simulink model "Posture_Regulation_NO_Singularity_ROS"  (R2022b)
settings: Solver=FixedStepAuto  StartTime=0.0  StopTime=80  FixedStep=0.02  MaxStep=0.1  RelTol=1e-3
undefined symbols (not defined in the file): theta_f, unicycle, X, x_f, Y, y_f
libraries: simulink_extras x4, robotlib x3
settings Model: Creator=Musta  LastModifiedBy=mustacchim
settings OptimizationCC: EnhancedBackFolding=on  PassReuseOutputArgsAs=Individual arguments  ZeroExternalMemoryAtStartup=off  ZeroInternalMemoryAtStartup=off  MaxStackSize=64  OptimizeBlockOrder=speed  DifferentSizesBufferReuse=on  OptimizationCustomize=off  EfficientTunableParamExpr=on
settings DebuggingCC: ParameterTunabilityLossMsg=error
settings HardwareCC: ProdBitPerPointer=32  ProdBitPerSizeT=32  ProdBitPerPtrDiffT=32  ProdLargestAtomicFloat=None  ProdIntDivRoundTo=Undefined  ProdEndianess=Unspecified  ProdWordSize=32  ProdHWDeviceType=Generic->Unspecified (assume 32-bit Generic)
settings SFSimCC: MATLABDynamicMemAlloc=off
settings RTWCC: Description=Embedded Coder  SystemTargetFile=ert.tlc  HardwareBoard=Robot Operating System (ROS)  TLCOptions="-aInlineSetEventsForThisBaseRateFcn=TLC_FALSE -aSuppressMultiTaskScheduler=TLC_FALSE  -aRateBasedStepFcn=0"  TemplateMakefile=ert_default_tmf  Toolchain=Catkin  TargetLang=C++
settings CodeAppCC: ForceParamTrailComments=on  IgnoreCustomStorageClasses=off  OperatorAnnotations=on  SimulinkDataObjDesc=on  SFDataObjDesc=on  InsertBlockDesc=on

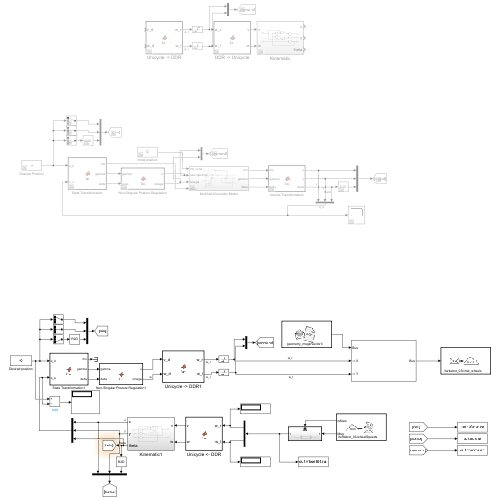
[thumbnail: Simulink's stored preview of the top-level diagram]
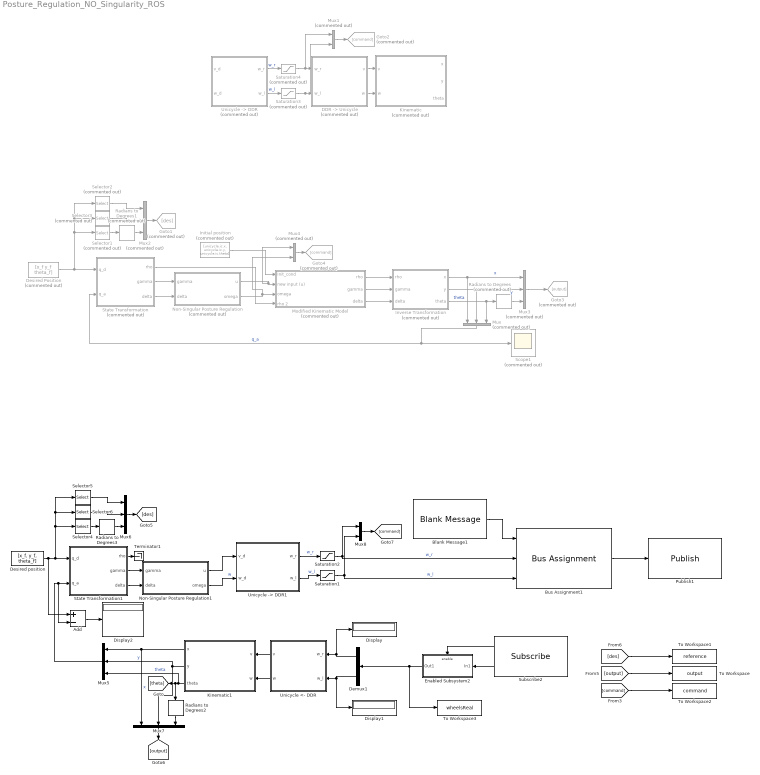
== system Posture_Regulation_NO_Singularity_ROS ==
  " DDR -> Unicycle " : MATLAB Function  Commented=on  TreatAsAtomicUnit=on
  Add : Sum  Inputs=+-
  Blank Message1 : robotlib/Blank Message  messageClass=Message  entityType=geometry_msgs/Vector3  messageType=geometry_msgs/Vector3  SampleTime=0.02  legacyBusStruct=off
      settings: LibrarySourceBlock=roslib/ROS/Blank Message
  Bus Assignment1 : BusAssignment  AssignedSignals=X,Y
  Demux1 : Demux  Outputs=2
  Desired Position : Constant  Commented=on  Value=[x_f y_f theta_f]
  Desired position : Constant  Value=[x_f, y_f, theta_f]
  Display : Display
  Display1 : Display
  Display2 : Display
  Enabled Subsystem2 : Subsystem  TreatAsAtomicUnit=on
  Goto1 : Goto  Commented=on  GotoTag=des
  Goto2 : Goto  Commented=on  GotoTag=command
  Goto3 : Goto  Commented=on  GotoTag=output
  Goto4 : Goto  Commented=on  GotoTag=command
  Initial position : Constant  Commented=on  Value=[unicycle.ic.x, unicycle.ic.y, unicycle.ic.theta]
  Inverse Transformation : MATLAB Function  Commented=on  TreatAsAtomicUnit=on
  Kinematic : Subsystem  Commented=on
  Kinematic1 : Subsystem
  Modified Kinematic Model : Subsystem  Commented=on
  Mux : Mux  Commented=on  Inputs=3
  Mux1 : Mux  Commented=on  Inputs=2
  Mux2 : Mux  Commented=on  Inputs=3
  Mux3 : Mux  Commented=on  Inputs=3
  Mux4 : Mux  Commented=on  Inputs=2
  Mux5 : Mux  Inputs=3
  Mux6 : Mux  Inputs=3
  Mux7 : Mux  Inputs=3
  Mux8 : Mux  Inputs=2
  Non-Singular Posture Regulation : MATLAB Function  Commented=on  TreatAsAtomicUnit=on
  Non-Singular Posture Regulation1 : MATLAB Function  TreatAsAtomicUnit=on
  Publish1 : robotlib/Publish  topicSource=Select from ROS network  topic=/turtlebot_03/cmd_wheels  messageType=geometry_msgs/Vector3  legacyBusStruct=off  messageQueueLength=1
      settings: LibrarySourceBlock=roslib/ROS/Publish
  Radians to Degrees : simulink_extras/Transformations/Radians to Degrees  Commented=on
  Radians to Degrees1 : simulink_extras/Transformations/Radians to Degrees  Commented=on
  Radians to Degrees2 : simulink_extras/Transformations/Radians to Degrees
  Radians to Degrees3 : simulink_extras/Transformations/Radians to Degrees
  Saturation1 : Saturate  UpperLimit=unicycle.omegaWheelMax  LowerLimit=unicycle.omegaWheelMin
  Saturation2 : Saturate  UpperLimit=unicycle.omegaWheelMax  LowerLimit=unicycle.omegaWheelMin
  Saturation3 : Saturate  Commented=on  UpperLimit=unicycle.omegaWheelMax  LowerLimit=unicycle.omegaWheelMin
  Saturation4 : Saturate  Commented=on  UpperLimit=unicycle.omegaWheelMax  LowerLimit=unicycle.omegaWheelMin
  Scope1 : Scope  Commented=on
  Selector1 : Selector  Commented=on  InputPortWidth=3  IndexOptions=Index vector (dialog)  Indices=3  OutputSizes=1
  Selector2 : Selector  Commented=on  InputPortWidth=3  IndexOptions=Index vector (dialog)  Indices=1  OutputSizes=1
  Selector3 : Selector  Commented=on  InputPortWidth=3  IndexOptions=Index vector (dialog)  Indices=2  OutputSizes=1
  Selector4 : Selector  InputPortWidth=3  IndexOptions=Index vector (dialog)  Indices=3  OutputSizes=1
  Selector5 : Selector  InputPortWidth=3  IndexOptions=Index vector (dialog)  Indices=1  OutputSizes=1
  Selector6 : Selector  InputPortWidth=3  IndexOptions=Index vector (dialog)  Indices=2  OutputSizes=1
  State Transformation : MATLAB Function  Commented=on  TreatAsAtomicUnit=on
  State Transformation1 : MATLAB Function  TreatAsAtomicUnit=on
  Subscribe2 : robotlib/Subscribe  topicSource=Select from ROS network  topic=/turtlebot_03/wheelSpeeds  messageType=geometry_msgs/Vector3  SampleTime=0.02  legacyBusStruct=off  messageQueueLength=1
      settings: LibrarySourceBlock=roslib/ROS/Subscribe
  Terminator1 : Terminator
  To Workspace : ToWorkspace  VariableName=output  SaveFormat=Structure With Time  SampleTime=-1
  To Workspace1 : ToWorkspace  VariableName=reference  SaveFormat=Structure With Time  SampleTime=-1
  To Workspace2 : ToWorkspace  VariableName=command  SaveFormat=Structure With Time  SampleTime=-1
  To Workspace3 : ToWorkspace  VariableName=wheelsReal  SaveFormat=Structure With Time  SampleTime=-1
  "Unicycle -> DDR" : MATLAB Function  Commented=on  TreatAsAtomicUnit=on
  "Unicycle -> DDR1" : MATLAB Function  TreatAsAtomicUnit=on
  Unicycle <- DDR : MATLAB Function  TreatAsAtomicUnit=on
  wires:
  [command] -> To Workspace2/1
  [des] -> To Workspace1/1
  [output] -> To Workspace/1
  Selector2/1 -> Mux2/1
  Mux/1 -> Scope1/1, State Transformation/2(q_a)  "q_a"
  Selector3/1 -> Mux2/2
  Inverse Transformation/1(x) -> Mux/1, Mux3/1  "x"
  Desired Position/1 -> Selector2/1, Selector3/1, Selector1/1, State Transformation/1(q_d)
  Inverse Transformation/3(theta) -> Mux/3, Radians to Degrees/1  "theta"
  Radians to Degrees/1 -> Mux3/3
  Inverse Transformation/2(y) -> Mux3/2, Mux/2  "y"
  Modified Kinematic Model/3(delta) -> Inverse Transformation/3(delta)
  Mux2/1 -> Goto1/1
  State Transformation/1(rho) -> Modified Kinematic Model/4(rho 2)
  Radians to Degrees1/1 -> Mux2/3
  Selector1/1 -> Radians to Degrees1/1
  Modified Kinematic Model/1(rho) -> Inverse Transformation/1(rho)
  Mux4/1 -> Goto4/1
  Modified Kinematic Model/2(gamma) -> Inverse Transformation/2(gamma)
  State Transformation/3(delta) -> Non-Singular Posture Regulation/2(delta)
  Initial position/1 -> Modified Kinematic Model/1(Init_cond)
  Non-Singular Posture Regulation/1(u) -> Modified Kinematic Model/2(new input (u)), Mux4/1
  Mux3/1 -> Goto3/1
  Non-Singular Posture Regulation/2(omega) -> Mux4/2, Modified Kinematic Model/3(omega)
  State Transformation/2(gamma) -> Non-Singular Posture Regulation/1(gamma)
  "Unicycle -> DDR"/2(w_l) -> Saturation3/1  "w_l"
  " DDR -> Unicycle "/1(v) -> Kinematic/1(v)
  "Unicycle -> DDR"/1(w_r) -> Saturation4/1  "w_r"
  Mux1/1 -> Goto2/1
  Saturation4/1 -> Mux1/1, " DDR -> Unicycle "/1(w_r)
  Saturation3/1 -> Mux1/2, " DDR -> Unicycle "/2(w_l)
  " DDR -> Unicycle "/2(w) -> Kinematic/2(w)
  Radians to Degrees2/1 -> Mux7/3
  Bus Assignment1/1 -> Publish1/1
  Selector4/1 -> Radians to Degrees3/1
  Subscribe2/2 -> Enabled Subsystem2/1(In1)
  State Transformation1/2(gamma) -> Non-Singular Posture Regulation1/1(gamma)
  Demux1/2 -> Display1/1, Unicycle <- DDR/2(w_l)
  Saturation2/1 -> Bus Assignment1/2, Mux8/1  "w_r"
  Unicycle <- DDR/1(v) -> Kinematic1/1(v)
  Mux6/1 -> [des]
  "Unicycle -> DDR1"/1(w_r) -> Saturation2/1  "w_r"
  Non-Singular Posture Regulation1/1(u) -> "Unicycle -> DDR1"/1(v_d)
  Kinematic1/3(theta) -> Mux5/3, Radians to Degrees2/1, [theta]  "theta"
  Saturation1/1 -> Bus Assignment1/3, Mux8/2  "w_l"
  State Transformation1/1(rho) -> Terminator1/1
  Demux1/1 -> Display/1, Unicycle <- DDR/1(w_r)
  Selector6/1 -> Mux6/2
  Mux7/1 -> [output]
  "Unicycle -> DDR1"/2(w_l) -> Saturation1/1  "w_l"
  Radians to Degrees3/1 -> Mux6/3
  Blank Message1/1 -> Bus Assignment1/1
  Kinematic1/2(y) -> Mux7/2, Mux5/2  "y"
  Unicycle <- DDR/2(w) -> Kinematic1/2(w)
  Mux5/1 -> Add/2, State Transformation1/2(q_a)
  Non-Singular Posture Regulation1/2(omega) -> "Unicycle -> DDR1"/2(w_d)  "w"
  Selector5/1 -> Mux6/1
  State Transformation1/3(delta) -> Non-Singular Posture Regulation1/2(delta)
  Enabled Subsystem2/1(Out1) -> To Workspace3/1, Demux1/1
  Mux8/1 -> [command]
  Kinematic1/1(x) -> Mux5/1, Mux7/1  "x"
  Subscribe2/1 -> Enabled Subsystem2/Enable
  Add/1 -> Display2/1
  Desired position/1 -> Add/1, State Transformation1/1(q_d), Selector5/1, Selector6/1, Selector4/1

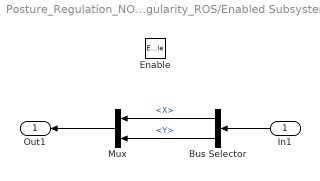
== system Posture_Regulation_NO_Singularity_ROS/Enabled Subsystem2 ==
  In1 : Inport
  Enable : EnablePort
  Bus Selector : BusSelector  OutputSignals=X,Y
  Mux : Mux  Inputs=2
  Out1 : Outport
  wires:
  Mux/1 -> Out1/1
  Bus Selector/1 -> Mux/1  "<X>"
  Bus Selector/2 -> Mux/2  "<Y>"
  In1/1 -> Bus Selector/1

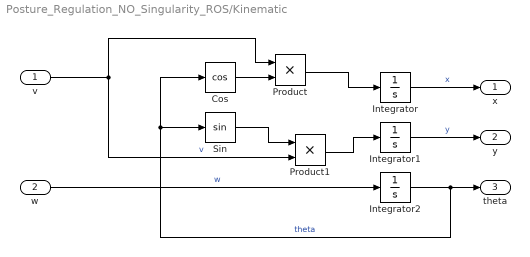
== system Posture_Regulation_NO_Singularity_ROS/Kinematic ==
  v : Inport
  w : Inport  Port=2
  Cos : Trigonometry  Operator=cos
  Integrator : Integrator  InitialCondition=unicycle.ic.x
  Integrator1 : Integrator  InitialCondition=unicycle.ic.y
  Integrator2 : Integrator  InitialCondition=unicycle.ic.theta
  Product : Product
  Product1 : Product
  Sin : Trigonometry
  x : Outport
  y : Outport  Port=2
  theta : Outport  Port=3
  wires:
  w/1 -> Integrator2/1  "w"
  Product/1 -> Integrator/1
  v/1 -> Product/1, Product1/2  "v"
  Cos/1 -> Product/2
  Integrator1/1 -> y/1  "y"
  Integrator/1 -> x/1  "x"
  Integrator2/1 -> Cos/1, Sin/1, theta/1  "theta"
  Product1/1 -> Integrator1/1
  Sin/1 -> Product1/1

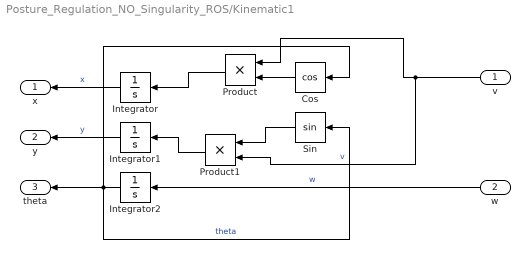
== system Posture_Regulation_NO_Singularity_ROS/Kinematic1 ==
  v : Inport
  w : Inport  Port=2
  Cos : Trigonometry  Operator=cos
  Integrator : Integrator  InitialCondition=unicycle.ic.x
  Integrator1 : Integrator  InitialCondition=unicycle.ic.y
  Integrator2 : Integrator  InitialCondition=unicycle.ic.theta
  Product : Product
  Product1 : Product
  Sin : Trigonometry
  x : Outport
  y : Outport  Port=2
  theta : Outport  Port=3
  wires:
  w/1 -> Integrator2/1  "w"
  Product/1 -> Integrator/1
  v/1 -> Product/1, Product1/2  "v"
  Cos/1 -> Product/2
  Integrator1/1 -> y/1  "y"
  Integrator/1 -> x/1  "x"
  Integrator2/1 -> theta/1, Sin/1, Cos/1  "theta"
  Product1/1 -> Integrator1/1
  Sin/1 -> Product1/1

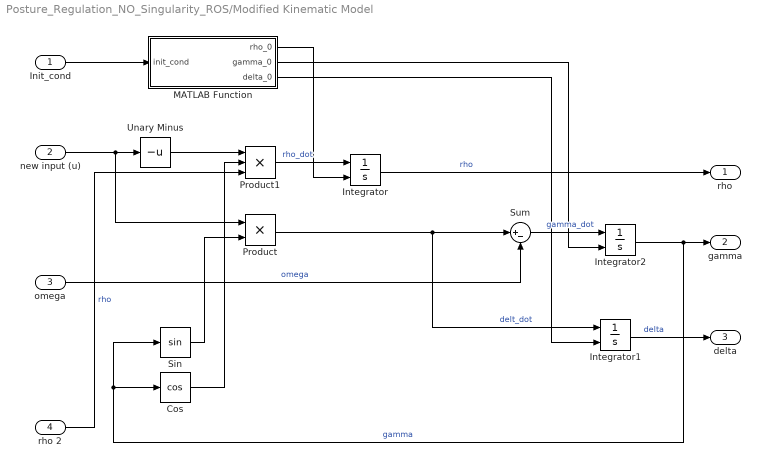
== system Posture_Regulation_NO_Singularity_ROS/Modified Kinematic Model ==
  Init_cond : Inport
  new input (u) : Inport  Port=2
  omega : Inport  Port=3
  rho 2 : Inport  Port=4
  Cos : Trigonometry  Operator=cos
  Integrator : Integrator  InitialConditionSource=external  InitialCondition=-10
  Integrator1 : Integrator  InitialConditionSource=external
  Integrator2 : Integrator  InitialConditionSource=external
  MATLAB Function : MATLAB Function  TreatAsAtomicUnit=on
  Product : Product
  Product1 : Product  Inputs=3
  Sin : Trigonometry
  Sum : Sum  Inputs=|+-
  Unary Minus : UnaryMinus
  rho : Outport
  gamma : Outport  Port=2
  delta : Outport  Port=3
  wires:
  Sum/1 -> Integrator2/1  "gamma_dot"
  Cos/1 -> Product1/2
  Unary Minus/1 -> Product1/1
  new input (u)/1 -> Product/1, Unary Minus/1
  Product1/1 -> Integrator/1  "rho_dot"
  Integrator/1 -> rho/1  "rho"
  Sin/1 -> Product/2
  Product/1 -> Sum/1, Integrator1/1  "delt_dot"
  omega/1 -> Sum/2  "omega"
  Integrator2/1 -> gamma/1, Cos/1, Sin/1  "gamma"
  Integrator1/1 -> delta/1  "delta"
  rho 2/1 -> Product1/3  "rho"
  Init_cond/1 -> MATLAB Function/1(init_cond)
  MATLAB Function/2(gamma_0) -> Integrator2/2
  MATLAB Function/3(delta_0) -> Integrator1/2
  MATLAB Function/1(rho_0) -> Integrator/2

== matlab function Posture_Regulation_NO_Singularity_ROS/ DDR -> Unicycle  ==
  data: w_r input; v output; w_l input; w output
function [v, w] = fcn(w_r, w_l)

    %#codegen
    coder.extrinsic('evalin')
    d = 0;                  % Needed in order to set variable class correctly
    r = 0;                  % Needed in order to set variable class correctly
    d = evalin('base','unicycle.d'); % Read value from workspace
    r = evalin('base','unicycle.r'); % Read value from workspace

    v = r*(w_r + w_l)/2; % rad/s
    w = r*(w_r - w_l)/d; % rad/s

end

== matlab function Posture_Regulation_NO_Singularity_ROS/Non-Singular Posture Regulation1 ==
  data: u output; omega output; gamma input; delta input
function [u,omega] = fcn(gamma,delta)

    %#codegen
    coder.extrinsic('evalin')
    k1 = 0;                  % Needed in order to set variable class correctly
    k2 = 0;                  % Needed in order to set variable class correctly
    k3 = 0;                  % Needed in order to set variable class correctly
    k1 = evalin('base','k1'); % Read value from workspace
    k2 = evalin('base','k2'); % Read value from workspace
    k3 = evalin('base','k3'); % Read value from workspace

    u = k1 * cos(gamma);
    omega = k2 * gamma + (k1 * sin(gamma)*cos(gamma)/gamma * (gamma + k3 * delta));

end

== matlab function Posture_Regulation_NO_Singularity_ROS/State Transformation1 ==
  data: q_d input; rho output; q_a input; gamma output; delta output
function [rho,gamma,delta] = fcn(q_d, q_a)

%     e_x = q_d(1) - q_a(1);
%     e_y = q_d(2) - q_a(2);
%     e_theta = q_d(3) - q_a(3);
%     
%     rho = sqrt(e_x^2 + e_y^2);
%     gamma = mod(atan2(e_y,e_x),2*pi) - q_a(3);
%     delta = gamma - e_theta;

    e_x = q_d(1) - q_a(1);
    e_y = q_d(2) - q_a(2);
    e_theta = q_d(3) - q_a(3);
   
    rho = sqrt(e_x^2 + e_y^2);

    p = atan2(e_y,e_x);
    % Count the number of turns around full circle
    num_turns = floor(p/(2*pi));
    % Adjust p to remove any full circle turns
    theta_adj = p - num_turns*(2*pi);

    % gamma = mod(theta_adj,2*pi) - q_a(3);
    gamma = theta_adj - q_a(3);
    delta = gamma - e_theta;

end

== matlab function Posture_Regulation_NO_Singularity_ROS/Unicycle -> DDR1 ==
  data: v_d input; w_r output; w_d input; w_l output
function [w_r, w_l] = fcn(v_d, w_d)

    %#codegen
    coder.extrinsic('evalin')
    d = 0;                  % Needed in order to set variable class correctly
    r = 0;                  % Needed in order to set variable class correctly
    d = evalin('base','unicycle.d'); % Read value from workspace
    r = evalin('base','unicycle.r'); % Read value from workspace

    w_r = ((2 * v_d) + (w_d * d)) / (2 * r);
    w_l = ((2 * v_d) - (w_d * d)) / (2 * r);

end

== matlab function Posture_Regulation_NO_Singularity_ROS/Non-Singular Posture Regulation ==
  data: u output; omega output; gamma input; delta input
function [u,omega] = fcn(gamma,delta)

    %#codegen
    coder.extrinsic('evalin')
    k1 = 0;                  % Needed in order to set variable class correctly
    k2 = 0;                  % Needed in order to set variable class correctly
    k3 = 0;                  % Needed in order to set variable class correctly
    k1 = evalin('base','k1'); % Read value from workspace
    k2 = evalin('base','k2'); % Read value from workspace
    k3 = evalin('base','k3'); % Read value from workspace

    u = k1 * cos(gamma);
    omega = k2 * gamma + (k1 * sin(gamma)*cos(gamma)/gamma * (gamma + k3 * delta));

end

== matlab function Posture_Regulation_NO_Singularity_ROS/State Transformation ==
  data: q_d input; rho output; q_a input; gamma output; delta output
function [rho,gamma,delta] = fcn(q_d, q_a)

    e_x = q_d(1) - q_a(1);
    e_y = q_d(2) - q_a(2);
    e_theta = q_d(3) - q_a(3);
    
    rho = sqrt(e_x^2 + e_y^2);
    gamma = mod(atan2(e_y,e_x),2*pi) - q_a(3);
    delta = gamma - e_theta;

end

== matlab function Posture_Regulation_NO_Singularity_ROS/Inverse Transformation ==
  data: x output; rho input; y output; gamma input; delta input; theta output
function [x,y,theta] = fcn(rho,gamma,delta)

    x = - rho * cos(delta);
    y = - rho * sin(delta);
    theta = delta - gamma;
    
end

== matlab function Posture_Regulation_NO_Singularity_ROS/Modified Kinematic Model/MATLAB Function ==
  data: init_cond input; rho_0 output; gamma_0 output; delta_0 output
function [rho_0, gamma_0, delta_0] = fcn(init_cond)

x_0 = init_cond(1);
y_0 = init_cond(2);
theta_0 = init_cond(3);


rho_0 = sqrt(x_0^2 + y_0^2);
gamma_0 = atan2(y_0,x_0) - theta_0 + pi;
delta_0 = gamma_0 + theta_0;

== matlab function Posture_Regulation_NO_Singularity_ROS/Unicycle <- DDR ==
  data: w_r input; v output; w_l input; w output
function [v, w] = fcn(w_r, w_l)

    %#codegen
    coder.extrinsic('evalin')
    d = 0;                  % Needed in order to set variable class correctly
    r = 0;                  % Needed in order to set variable class correctly
    d = evalin('base','unicycle.d'); % Read value from workspace
    r = evalin('base','unicycle.r'); % Read value from workspace

    v = r*(w_r + w_l)/2; % rad/s
    w = r*(w_r - w_l)/d; % rad/s

end

== matlab function Posture_Regulation_NO_Singularity_ROS/Unicycle -> DDR ==
  data: v_d input; w_r output; w_d input; w_l output
function [w_r, w_l] = fcn(v_d, w_d)

    %#codegen
    coder.extrinsic('evalin')
    d = 0;                  % Needed in order to set variable class correctly
    r = 0;                  % Needed in order to set variable class correctly
    d = evalin('base','unicycle.d'); % Read value from workspace
    r = evalin('base','unicycle.r'); % Read value from workspace

    w_r = ((2 * v_d) + (w_d * d)) / (2 * r);
    w_l = ((2 * v_d) - (w_d * d)) / (2 * r);

end
